simulink model "reduce_spect"  (R2013b)
settings: Solver=ode45  StartTime=0.0  StopTime=10.0  RelTol=1e-3
undefined symbols (not defined in the file): pfb_coeff_gen_calc
libraries: xbsIndex_r4 x15467, casper_library_delays x101, casper_library_misc x85, dspsigops x16, xps_library x4, xbsReplacements_r4 x2, casper_library_pfbs x2
(part 6 of 157)

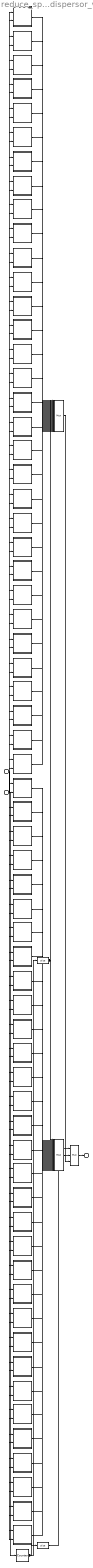
== system reduce_spect/Dedispersor_v4 ==
  Data : Inport
  Valid : Inport  Port=2
  Counter : xbsIndex_r4/Counter  cnt_type=Free Running  cnt_to=Inf  operation=Up  start_count=0  cnt_by_val=1  arith_type=Unsigned  n_bits=6  bin_pt=0  load_pin=off  rst=off  en=on  explicit_period=on  period=1  dbl_ovrd=off  use_behavioral_HDL=off  implementation=Fabric  block_type=counter
  Mux : xbsIndex_r4/Mux  inputs=32  en=off  latency=0  precision=Full  arith_type=Unsigned  n_bits=16  bin_pt=14  quantization=Truncate  overflow=Wrap  dbl_ovrd=off  block_type=mux
  Mux1 : xbsIndex_r4/Mux  inputs=32  en=off  latency=0  precision=Full  arith_type=Unsigned  n_bits=16  bin_pt=14  quantization=Truncate  overflow=Wrap  dbl_ovrd=off  block_type=mux
  Mux2 : xbsIndex_r4/Mux  inputs=2  en=off  latency=0  precision=Full  arith_type=Unsigned  n_bits=16  bin_pt=14  quantization=Truncate  overflow=Wrap  dbl_ovrd=off  block_type=mux
  Slice : xbsIndex_r4/Slice  nbits=5  boolean_output=off  mode=Lower Bit Location + Width  bit1=0  base1=MSB of Input  bit0=0  base0=LSB of Input  dbl_ovrd=off  block_type=slice
  Slice1 : xbsIndex_r4/Slice  nbits=1  boolean_output=off  mode=Upper Bit Location + Width  bit1=0  base1=MSB of Input  bit0=0  base0=LSB of Input  dbl_ovrd=off  block_type=slice
  detector_block_v2 : Subsystem  AncestorBlock=honestlibrary/detector_block_v2  mask(Basic block for FRB detection){chn=0, lat=1, nbits=6, behavioral=on}
      mask prompts: chn "Channel"; lat "Latency"; nbits "Number of Bits (Counter)"; behavioral "behavioral delay"
      mask help:
      | Delays a certain channel a number of latency clock cycles, according to the fixed DM table.
      | This version incorporates an internal counter (nbits) to know when store or give a certain value.
      mask init:
      | detector_block_init_v2(gcb,'chn',chn,'lat',lat,'nbits',nbits,'behavioral', behavioral)
      settings: AttributesFormatString=Channel: 0, Delay: 1
  detector_block_v21 : Subsystem  AncestorBlock=honestlibrary/detector_block_v2  mask(Basic block for FRB detection){chn=1, lat=2, nbits=6, behavioral=on}
      mask prompts: chn "Channel"; lat "Latency"; nbits "Number of Bits (Counter)"; behavioral "behavioral delay"
      mask help:
      | Delays a certain channel a number of latency clock cycles, according to the fixed DM table.
      | This version incorporates an internal counter (nbits) to know when store or give a certain value.
      mask init:
      | detector_block_init_v2(gcb,'chn',chn,'lat',lat,'nbits',nbits,'behavioral', behavioral)
      settings: AttributesFormatString=Channel: 1, Delay: 2
  detector_block_v210 : Subsystem  AncestorBlock=honestlibrary/detector_block_v2  mask(Basic block for FRB detection){chn=10, lat=29, nbits=6, behavioral=on}
      mask prompts: chn "Channel"; lat "Latency"; nbits "Number of Bits (Counter)"; behavioral "behavioral delay"
      mask help:
      | Delays a certain channel a number of latency clock cycles, according to the fixed DM table.
      | This version incorporates an internal counter (nbits) to know when store or give a certain value.
      mask init:
      | detector_block_init_v2(gcb,'chn',chn,'lat',lat,'nbits',nbits,'behavioral', behavioral)
      settings: AttributesFormatString=Channel: 10, Delay: 29
  detector_block_v211 : Subsystem  AncestorBlock=honestlibrary/detector_block_v2  mask(Basic block for FRB detection){chn=11, lat=31, nbits=6, behavioral=on}
      mask prompts: chn "Channel"; lat "Latency"; nbits "Number of Bits (Counter)"; behavioral "behavioral delay"
      mask help:
      | Delays a certain channel a number of latency clock cycles, according to the fixed DM table.
      | This version incorporates an internal counter (nbits) to know when store or give a certain value.
      mask init:
      | detector_block_init_v2(gcb,'chn',chn,'lat',lat,'nbits',nbits,'behavioral', behavioral)
      settings: AttributesFormatString=Channel: 11, Delay: 31
  detector_block_v212 : Subsystem  AncestorBlock=honestlibrary/detector_block_v2  mask(Basic block for FRB detection){chn=12, lat=34, nbits=6, behavioral=on}
      mask prompts: chn "Channel"; lat "Latency"; nbits "Number of Bits (Counter)"; behavioral "behavioral delay"
      mask help:
      | Delays a certain channel a number of latency clock cycles, according to the fixed DM table.
      | This version incorporates an internal counter (nbits) to know when store or give a certain value.
      mask init:
      | detector_block_init_v2(gcb,'chn',chn,'lat',lat,'nbits',nbits,'behavioral', behavioral)
      settings: AttributesFormatString=Channel: 12, Delay: 34
  detector_block_v213 : Subsystem  AncestorBlock=honestlibrary/detector_block_v2  mask(Basic block for FRB detection){chn=13, lat=37, nbits=6, behavioral=on}
      mask prompts: chn "Channel"; lat "Latency"; nbits "Number of Bits (Counter)"; behavioral "behavioral delay"
      mask help:
      | Delays a certain channel a number of latency clock cycles, according to the fixed DM table.
      | This version incorporates an internal counter (nbits) to know when store or give a certain value.
      mask init:
      | detector_block_init_v2(gcb,'chn',chn,'lat',lat,'nbits',nbits,'behavioral', behavioral)
      settings: AttributesFormatString=Channel: 13, Delay: 37
  detector_block_v214 : Subsystem  AncestorBlock=honestlibrary/detector_block_v2  mask(Basic block for FRB detection){chn=14, lat=39, nbits=6, behavioral=on}
      mask prompts: chn "Channel"; lat "Latency"; nbits "Number of Bits (Counter)"; behavioral "behavioral delay"
      mask help:
      | Delays a certain channel a number of latency clock cycles, according to the fixed DM table.
      | This version incorporates an internal counter (nbits) to know when store or give a certain value.
      mask init:
      | detector_block_init_v2(gcb,'chn',chn,'lat',lat,'nbits',nbits,'behavioral', behavioral)
      settings: AttributesFormatString=Channel: 14, Delay: 39
  detector_block_v215 : Subsystem  AncestorBlock=honestlibrary/detector_block_v2  mask(Basic block for FRB detection){chn=15, lat=41, nbits=6, behavioral=on}
      mask prompts: chn "Channel"; lat "Latency"; nbits "Number of Bits (Counter)"; behavioral "behavioral delay"
      mask help:
      | Delays a certain channel a number of latency clock cycles, according to the fixed DM table.
      | This version incorporates an internal counter (nbits) to know when store or give a certain value.
      mask init:
      | detector_block_init_v2(gcb,'chn',chn,'lat',lat,'nbits',nbits,'behavioral', behavioral)
      settings: AttributesFormatString=Channel: 15, Delay: 41
  detector_block_v216 : Subsystem  AncestorBlock=honestlibrary/detector_block_v2  mask(Basic block for FRB detection){chn=16, lat=44, nbits=6, behavioral=on}
      mask prompts: chn "Channel"; lat "Latency"; nbits "Number of Bits (Counter)"; behavioral "behavioral delay"
      mask help:
      | Delays a certain channel a number of latency clock cycles, according to the fixed DM table.
      | This version incorporates an internal counter (nbits) to know when store or give a certain value.
      mask init:
      | detector_block_init_v2(gcb,'chn',chn,'lat',lat,'nbits',nbits,'behavioral', behavioral)
      settings: AttributesFormatString=Channel: 16, Delay: 44
  detector_block_v217 : Subsystem  AncestorBlock=honestlibrary/detector_block_v2  mask(Basic block for FRB detection){chn=17, lat=46, nbits=6, behavioral=on}
      mask prompts: chn "Channel"; lat "Latency"; nbits "Number of Bits (Counter)"; behavioral "behavioral delay"
      mask help:
      | Delays a certain channel a number of latency clock cycles, according to the fixed DM table.
      | This version incorporates an internal counter (nbits) to know when store or give a certain value.
      mask init:
      | detector_block_init_v2(gcb,'chn',chn,'lat',lat,'nbits',nbits,'behavioral', behavioral)
      settings: AttributesFormatString=Channel: 17, Delay: 46
  detector_block_v218 : Subsystem  AncestorBlock=honestlibrary/detector_block_v2  mask(Basic block for FRB detection){chn=18, lat=48, nbits=6, behavioral=on}
      mask prompts: chn "Channel"; lat "Latency"; nbits "Number of Bits (Counter)"; behavioral "behavioral delay"
      mask help:
      | Delays a certain channel a number of latency clock cycles, according to the fixed DM table.
      | This version incorporates an internal counter (nbits) to know when store or give a certain value.
      mask init:
      | detector_block_init_v2(gcb,'chn',chn,'lat',lat,'nbits',nbits,'behavioral', behavioral)
      settings: AttributesFormatString=Channel: 18, Delay: 48
  detector_block_v219 : Subsystem  AncestorBlock=honestlibrary/detector_block_v2  mask(Basic block for FRB detection){chn=19, lat=51, nbits=6, behavioral=on}
      mask prompts: chn "Channel"; lat "Latency"; nbits "Number of Bits (Counter)"; behavioral "behavioral delay"
      mask help:
      | Delays a certain channel a number of latency clock cycles, according to the fixed DM table.
      | This version incorporates an internal counter (nbits) to know when store or give a certain value.
      mask init:
      | detector_block_init_v2(gcb,'chn',chn,'lat',lat,'nbits',nbits,'behavioral', behavioral)
      settings: AttributesFormatString=Channel: 19, Delay: 51
  detector_block_v22 : Subsystem  AncestorBlock=honestlibrary/detector_block_v2  mask(Basic block for FRB detection){chn=2, lat=5, nbits=6, behavioral=on}
      mask prompts: chn "Channel"; lat "Latency"; nbits "Number of Bits (Counter)"; behavioral "behavioral delay"
      mask help:
      | Delays a certain channel a number of latency clock cycles, according to the fixed DM table.
      | This version incorporates an internal counter (nbits) to know when store or give a certain value.
      mask init:
      | detector_block_init_v2(gcb,'chn',chn,'lat',lat,'nbits',nbits,'behavioral', behavioral)
      settings: AttributesFormatString=Channel: 2, Delay: 5
  detector_block_v220 : Subsystem  AncestorBlock=honestlibrary/detector_block_v2  mask(Basic block for FRB detection){chn=20, lat=53, nbits=6, behavioral=on}
      mask prompts: chn "Channel"; lat "Latency"; nbits "Number of Bits (Counter)"; behavioral "behavioral delay"
      mask help:
      | Delays a certain channel a number of latency clock cycles, according to the fixed DM table.
      | This version incorporates an internal counter (nbits) to know when store or give a certain value.
      mask init:
      | detector_block_init_v2(gcb,'chn',chn,'lat',lat,'nbits',nbits,'behavioral', behavioral)
      settings: AttributesFormatString=Channel: 20, Delay: 53
  detector_block_v221 : Subsystem  AncestorBlock=honestlibrary/detector_block_v2  mask(Basic block for FRB detection){chn=21, lat=55, nbits=6, behavioral=on}
      mask prompts: chn "Channel"; lat "Latency"; nbits "Number of Bits (Counter)"; behavioral "behavioral delay"
      mask help:
      | Delays a certain channel a number of latency clock cycles, according to the fixed DM table.
      | This version incorporates an internal counter (nbits) to know when store or give a certain value.
      mask init:
      | detector_block_init_v2(gcb,'chn',chn,'lat',lat,'nbits',nbits,'behavioral', behavioral)
      settings: AttributesFormatString=Channel: 21, Delay: 55
  detector_block_v222 : Subsystem  AncestorBlock=honestlibrary/detector_block_v2  mask(Basic block for FRB detection){chn=22, lat=57, nbits=6, behavioral=on}
      mask prompts: chn "Channel"; lat "Latency"; nbits "Number of Bits (Counter)"; behavioral "behavioral delay"
      mask help:
      | Delays a certain channel a number of latency clock cycles, according to the fixed DM table.
      | This version incorporates an internal counter (nbits) to know when store or give a certain value.
      mask init:
      | detector_block_init_v2(gcb,'chn',chn,'lat',lat,'nbits',nbits,'behavioral', behavioral)
      settings: AttributesFormatString=Channel: 22, Delay: 57
  detector_block_v223 : Subsystem  AncestorBlock=honestlibrary/detector_block_v2  mask(Basic block for FRB detection){chn=23, lat=59, nbits=6, behavioral=on}
      mask prompts: chn "Channel"; lat "Latency"; nbits "Number of Bits (Counter)"; behavioral "behavioral delay"
      mask help:
      | Delays a certain channel a number of latency clock cycles, according to the fixed DM table.
      | This version incorporates an internal counter (nbits) to know when store or give a certain value.
      mask init:
      | detector_block_init_v2(gcb,'chn',chn,'lat',lat,'nbits',nbits,'behavioral', behavioral)
      settings: AttributesFormatString=Channel: 23, Delay: 59
  detector_block_v224 : Subsystem  AncestorBlock=honestlibrary/detector_block_v2  mask(Basic block for FRB detection){chn=24, lat=61, nbits=6, behavioral=on}
      mask prompts: chn "Channel"; lat "Latency"; nbits "Number of Bits (Counter)"; behavioral "behavioral delay"
      mask help:
      | Delays a certain channel a number of latency clock cycles, according to the fixed DM table.
      | This version incorporates an internal counter (nbits) to know when store or give a certain value.
      mask init:
      | detector_block_init_v2(gcb,'chn',chn,'lat',lat,'nbits',nbits,'behavioral', behavioral)
      settings: AttributesFormatString=Channel: 24, Delay: 61
  detector_block_v225 : Subsystem  AncestorBlock=honestlibrary/detector_block_v2  mask(Basic block for FRB detection){chn=25, lat=63, nbits=6, behavioral=on}
      mask prompts: chn "Channel"; lat "Latency"; nbits "Number of Bits (Counter)"; behavioral "behavioral delay"
      mask help:
      | Delays a certain channel a number of latency clock cycles, according to the fixed DM table.
      | This version incorporates an internal counter (nbits) to know when store or give a certain value.
      mask init:
      | detector_block_init_v2(gcb,'chn',chn,'lat',lat,'nbits',nbits,'behavioral', behavioral)
      settings: AttributesFormatString=Channel: 25, Delay: 63
  detector_block_v226 : Subsystem  AncestorBlock=honestlibrary/detector_block_v2  mask(Basic block for FRB detection){chn=26, lat=65, nbits=6, behavioral=on}
      mask prompts: chn "Channel"; lat "Latency"; nbits "Number of Bits (Counter)"; behavioral "behavioral delay"
      mask help:
      | Delays a certain channel a number of latency clock cycles, according to the fixed DM table.
      | This version incorporates an internal counter (nbits) to know when store or give a certain value.
      mask init:
      | detector_block_init_v2(gcb,'chn',chn,'lat',lat,'nbits',nbits,'behavioral', behavioral)
      settings: AttributesFormatString=Channel: 26, Delay: 65
  detector_block_v227 : Subsystem  AncestorBlock=honestlibrary/detector_block_v2  mask(Basic block for FRB detection){chn=27, lat=67, nbits=6, behavioral=on}
      mask prompts: chn "Channel"; lat "Latency"; nbits "Number of Bits (Counter)"; behavioral "behavioral delay"
      mask help:
      | Delays a certain channel a number of latency clock cycles, according to the fixed DM table.
      | This version incorporates an internal counter (nbits) to know when store or give a certain value.
      mask init:
      | detector_block_init_v2(gcb,'chn',chn,'lat',lat,'nbits',nbits,'behavioral', behavioral)
      settings: AttributesFormatString=Channel: 27, Delay: 67
  detector_block_v228 : Subsystem  AncestorBlock=honestlibrary/detector_block_v2  mask(Basic block for FRB detection){chn=28, lat=69, nbits=6, behavioral=on}
      mask prompts: chn "Channel"; lat "Latency"; nbits "Number of Bits (Counter)"; behavioral "behavioral delay"
      mask help:
      | Delays a certain channel a number of latency clock cycles, according to the fixed DM table.
      | This version incorporates an internal counter (nbits) to know when store or give a certain value.
      mask init:
      | detector_block_init_v2(gcb,'chn',chn,'lat',lat,'nbits',nbits,'behavioral', behavioral)
      settings: AttributesFormatString=Channel: 28, Delay: 69
  detector_block_v229 : Subsystem  AncestorBlock=honestlibrary/detector_block_v2  mask(Basic block for FRB detection){chn=29, lat=71, nbits=6, behavioral=on}
      mask prompts: chn "Channel"; lat "Latency"; nbits "Number of Bits (Counter)"; behavioral "behavioral delay"
      mask help:
      | Delays a certain channel a number of latency clock cycles, according to the fixed DM table.
      | This version incorporates an internal counter (nbits) to know when store or give a certain value.
      mask init:
      | detector_block_init_v2(gcb,'chn',chn,'lat',lat,'nbits',nbits,'behavioral', behavioral)
      settings: AttributesFormatString=Channel: 29, Delay: 71
  detector_block_v23 : Subsystem  AncestorBlock=honestlibrary/detector_block_v2  mask(Basic block for FRB detection){chn=3, lat=8, nbits=6, behavioral=on}
      mask prompts: chn "Channel"; lat "Latency"; nbits "Number of Bits (Counter)"; behavioral "behavioral delay"
      mask help:
      | Delays a certain channel a number of latency clock cycles, according to the fixed DM table.
      | This version incorporates an internal counter (nbits) to know when store or give a certain value.
      mask init:
      | detector_block_init_v2(gcb,'chn',chn,'lat',lat,'nbits',nbits,'behavioral', behavioral)
      settings: AttributesFormatString=Channel: 3, Delay: 8
  detector_block_v230 : Subsystem  AncestorBlock=honestlibrary/detector_block_v2  mask(Basic block for FRB detection){chn=30, lat=73, nbits=6, behavioral=on}
      mask prompts: chn "Channel"; lat "Latency"; nbits "Number of Bits (Counter)"; behavioral "behavioral delay"
      mask help:
      | Delays a certain channel a number of latency clock cycles, according to the fixed DM table.
      | This version incorporates an internal counter (nbits) to know when store or give a certain value.
      mask init:
      | detector_block_init_v2(gcb,'chn',chn,'lat',lat,'nbits',nbits,'behavioral', behavioral)
      settings: AttributesFormatString=Channel: 30, Delay: 73
  detector_block_v231 : Subsystem  AncestorBlock=honestlibrary/detector_block_v2  mask(Basic block for FRB detection){chn=31, lat=74, nbits=6, behavioral=on}
      mask prompts: chn "Channel"; lat "Latency"; nbits "Number of Bits (Counter)"; behavioral "behavioral delay"
      mask help:
      | Delays a certain channel a number of latency clock cycles, according to the fixed DM table.
      | This version incorporates an internal counter (nbits) to know when store or give a certain value.
      mask init:
      | detector_block_init_v2(gcb,'chn',chn,'lat',lat,'nbits',nbits,'behavioral', behavioral)
      settings: AttributesFormatString=Channel: 31, Delay: 74
  detector_block_v232 : Subsystem  AncestorBlock=honestlibrary/detector_block_v2  mask(Basic block for FRB detection){chn=32, lat=76, nbits=6, behavioral=on}
      mask prompts: chn "Channel"; lat "Latency"; nbits "Number of Bits (Counter)"; behavioral "behavioral delay"
      mask help:
      | Delays a certain channel a number of latency clock cycles, according to the fixed DM table.
      | This version incorporates an internal counter (nbits) to know when store or give a certain value.
      mask init:
      | detector_block_init_v2(gcb,'chn',chn,'lat',lat,'nbits',nbits,'behavioral', behavioral)
      settings: AttributesFormatString=Channel: 32, Delay: 76
  detector_block_v233 : Subsystem  AncestorBlock=honestlibrary/detector_block_v2  mask(Basic block for FRB detection){chn=33, lat=78, nbits=6, behavioral=on}
      mask prompts: chn "Channel"; lat "Latency"; nbits "Number of Bits (Counter)"; behavioral "behavioral delay"
      mask help:
      | Delays a certain channel a number of latency clock cycles, according to the fixed DM table.
      | This version incorporates an internal counter (nbits) to know when store or give a certain value.
      mask init:
      | detector_block_init_v2(gcb,'chn',chn,'lat',lat,'nbits',nbits,'behavioral', behavioral)
      settings: AttributesFormatString=Channel: 33, Delay: 78
  detector_block_v234 : Subsystem  AncestorBlock=honestlibrary/detector_block_v2  mask(Basic block for FRB detection){chn=34, lat=79, nbits=6, behavioral=on}
      mask prompts: chn "Channel"; lat "Latency"; nbits "Number of Bits (Counter)"; behavioral "behavioral delay"
      mask help:
      | Delays a certain channel a number of latency clock cycles, according to the fixed DM table.
      | This version incorporates an internal counter (nbits) to know when store or give a certain value.
      mask init:
      | detector_block_init_v2(gcb,'chn',chn,'lat',lat,'nbits',nbits,'behavioral', behavioral)
      settings: AttributesFormatString=Channel: 34, Delay: 79
  detector_block_v235 : Subsystem  AncestorBlock=honestlibrary/detector_block_v2  mask(Basic block for FRB detection){chn=35, lat=81, nbits=6, behavioral=on}
      mask prompts: chn "Channel"; lat "Latency"; nbits "Number of Bits (Counter)"; behavioral "behavioral delay"
      mask help:
      | Delays a certain channel a number of latency clock cycles, according to the fixed DM table.
      | This version incorporates an internal counter (nbits) to know when store or give a certain value.
      mask init:
      | detector_block_init_v2(gcb,'chn',chn,'lat',lat,'nbits',nbits,'behavioral', behavioral)
      settings: AttributesFormatString=Channel: 35, Delay: 81
  detector_block_v236 : Subsystem  AncestorBlock=honestlibrary/detector_block_v2  mask(Basic block for FRB detection){chn=36, lat=83, nbits=6, behavioral=on}
      mask prompts: chn "Channel"; lat "Latency"; nbits "Number of Bits (Counter)"; behavioral "behavioral delay"
      mask help:
      | Delays a certain channel a number of latency clock cycles, according to the fixed DM table.
      | This version incorporates an internal counter (nbits) to know when store or give a certain value.
      mask init:
      | detector_block_init_v2(gcb,'chn',chn,'lat',lat,'nbits',nbits,'behavioral', behavioral)
      settings: AttributesFormatString=Channel: 36, Delay: 83
  detector_block_v237 : Subsystem  AncestorBlock=honestlibrary/detector_block_v2  mask(Basic block for FRB detection){chn=37, lat=84, nbits=6, behavioral=on}
      mask prompts: chn "Channel"; lat "Latency"; nbits "Number of Bits (Counter)"; behavioral "behavioral delay"
      mask help:
      | Delays a certain channel a number of latency clock cycles, according to the fixed DM table.
      | This version incorporates an internal counter (nbits) to know when store or give a certain value.
      mask init:
      | detector_block_init_v2(gcb,'chn',chn,'lat',lat,'nbits',nbits,'behavioral', behavioral)
      settings: AttributesFormatString=Channel: 37, Delay: 84
  detector_block_v238 : Subsystem  AncestorBlock=honestlibrary/detector_block_v2  mask(Basic block for FRB detection){chn=38, lat=86, nbits=6, behavioral=on}
      mask prompts: chn "Channel"; lat "Latency"; nbits "Number of Bits (Counter)"; behavioral "behavioral delay"
      mask help:
      | Delays a certain channel a number of latency clock cycles, according to the fixed DM table.
      | This version incorporates an internal counter (nbits) to know when store or give a certain value.
      mask init:
      | detector_block_init_v2(gcb,'chn',chn,'lat',lat,'nbits',nbits,'behavioral', behavioral)
      settings: AttributesFormatString=Channel: 38, Delay: 86
  detector_block_v239 : Subsystem  AncestorBlock=honestlibrary/detector_block_v2  mask(Basic block for FRB detection){chn=39, lat=87, nbits=6, behavioral=on}
      mask prompts: chn "Channel"; lat "Latency"; nbits "Number of Bits (Counter)"; behavioral "behavioral delay"
      mask help:
      | Delays a certain channel a number of latency clock cycles, according to the fixed DM table.
      | This version incorporates an internal counter (nbits) to know when store or give a certain value.
      mask init:
      | detector_block_init_v2(gcb,'chn',chn,'lat',lat,'nbits',nbits,'behavioral', behavioral)
      settings: AttributesFormatString=Channel: 39, Delay: 87
  detector_block_v24 : Subsystem  AncestorBlock=honestlibrary/detector_block_v2  mask(Basic block for FRB detection){chn=4, lat=12, nbits=6, behavioral=on}
      mask prompts: chn "Channel"; lat "Latency"; nbits "Number of Bits (Counter)"; behavioral "behavioral delay"
      mask help:
      | Delays a certain channel a number of latency clock cycles, according to the fixed DM table.
      | This version incorporates an internal counter (nbits) to know when store or give a certain value.
      mask init:
      | detector_block_init_v2(gcb,'chn',chn,'lat',lat,'nbits',nbits,'behavioral', behavioral)
      settings: AttributesFormatString=Channel: 4, Delay: 12
  detector_block_v240 : Subsystem  AncestorBlock=honestlibrary/detector_block_v2  mask(Basic block for FRB detection){chn=40, lat=89, nbits=6, behavioral=on}
      mask prompts: chn "Channel"; lat "Latency"; nbits "Number of Bits (Counter)"; behavioral "behavioral delay"
      mask help:
      | Delays a certain channel a number of latency clock cycles, according to the fixed DM table.
      | This version incorporates an internal counter (nbits) to know when store or give a certain value.
      mask init:
      | detector_block_init_v2(gcb,'chn',chn,'lat',lat,'nbits',nbits,'behavioral', behavioral)
      settings: AttributesFormatString=Channel: 40, Delay: 89
  detector_block_v241 : Subsystem  AncestorBlock=honestlibrary/detector_block_v2  mask(Basic block for FRB detection){chn=41, lat=90, nbits=6, behavioral=on}
      mask prompts: chn "Channel"; lat "Latency"; nbits "Number of Bits (Counter)"; behavioral "behavioral delay"
      mask help:
      | Delays a certain channel a number of latency clock cycles, according to the fixed DM table.
      | This version incorporates an internal counter (nbits) to know when store or give a certain value.
      mask init:
      | detector_block_init_v2(gcb,'chn',chn,'lat',lat,'nbits',nbits,'behavioral', behavioral)
      settings: AttributesFormatString=Channel: 41, Delay: 90
  detector_block_v242 : Subsystem  AncestorBlock=honestlibrary/detector_block_v2  mask(Basic block for FRB detection){chn=42, lat=92, nbits=6, behavioral=on}
      mask prompts: chn "Channel"; lat "Latency"; nbits "Number of Bits (Counter)"; behavioral "behavioral delay"
      mask help:
      | Delays a certain channel a number of latency clock cycles, according to the fixed DM table.
      | This version incorporates an internal counter (nbits) to know when store or give a certain value.
      mask init:
      | detector_block_init_v2(gcb,'chn',chn,'lat',lat,'nbits',nbits,'behavioral', behavioral)
      settings: AttributesFormatString=Channel: 42, Delay: 92
  detector_block_v243 : Subsystem  AncestorBlock=honestlibrary/detector_block_v2  mask(Basic block for FRB detection){chn=43, lat=93, nbits=6, behavioral=on}
      mask prompts: chn "Channel"; lat "Latency"; nbits "Number of Bits (Counter)"; behavioral "behavioral delay"
      mask help:
      | Delays a certain channel a number of latency clock cycles, according to the fixed DM table.
      | This version incorporates an internal counter (nbits) to know when store or give a certain value.
      mask init:
      | detector_block_init_v2(gcb,'chn',chn,'lat',lat,'nbits',nbits,'behavioral', behavioral)
      settings: AttributesFormatString=Channel: 43, Delay: 93
  detector_block_v244 : Subsystem  AncestorBlock=honestlibrary/detector_block_v2  mask(Basic block for FRB detection){chn=44, lat=95, nbits=6, behavioral=on}
      mask prompts: chn "Channel"; lat "Latency"; nbits "Number of Bits (Counter)"; behavioral "behavioral delay"
      mask help:
      | Delays a certain channel a number of latency clock cycles, according to the fixed DM table.
      | This version incorporates an internal counter (nbits) to know when store or give a certain value.
      mask init:
      | detector_block_init_v2(gcb,'chn',chn,'lat',lat,'nbits',nbits,'behavioral', behavioral)
      settings: AttributesFormatString=Channel: 44, Delay: 95
  detector_block_v245 : Subsystem  AncestorBlock=honestlibrary/detector_block_v2  mask(Basic block for FRB detection){chn=45, lat=96, nbits=6, behavioral=on}
      mask prompts: chn "Channel"; lat "Latency"; nbits "Number of Bits (Counter)"; behavioral "behavioral delay"
      mask help:
      | Delays a certain channel a number of latency clock cycles, according to the fixed DM table.
      | This version incorporates an internal counter (nbits) to know when store or give a certain value.
      mask init:
      | detector_block_init_v2(gcb,'chn',chn,'lat',lat,'nbits',nbits,'behavioral', behavioral)
      settings: AttributesFormatString=Channel: 45, Delay: 96
  detector_block_v246 : Subsystem  AncestorBlock=honestlibrary/detector_block_v2  mask(Basic block for FRB detection){chn=46, lat=97, nbits=6, behavioral=on}
      mask prompts: chn "Channel"; lat "Latency"; nbits "Number of Bits (Counter)"; behavioral "behavioral delay"
      mask help:
      | Delays a certain channel a number of latency clock cycles, according to the fixed DM table.
      | This version incorporates an internal counter (nbits) to know when store or give a certain value.
      mask init:
      | detector_block_init_v2(gcb,'chn',chn,'lat',lat,'nbits',nbits,'behavioral', behavioral)
      settings: AttributesFormatString=Channel: 46, Delay: 97
  detector_block_v247 : Subsystem  AncestorBlock=honestlibrary/detector_block_v2  mask(Basic block for FRB detection){chn=47, lat=99, nbits=6, behavioral=on}
      mask prompts: chn "Channel"; lat "Latency"; nbits "Number of Bits (Counter)"; behavioral "behavioral delay"
      mask help:
      | Delays a certain channel a number of latency clock cycles, according to the fixed DM table.
      | This version incorporates an internal counter (nbits) to know when store or give a certain value.
      mask init:
      | detector_block_init_v2(gcb,'chn',chn,'lat',lat,'nbits',nbits,'behavioral', behavioral)
      settings: AttributesFormatString=Channel: 47, Delay: 99
  detector_block_v248 : Subsystem  AncestorBlock=honestlibrary/detector_block_v2  mask(Basic block for FRB detection){chn=48, lat=100, nbits=6, behavioral=on}
      mask prompts: chn "Channel"; lat "Latency"; nbits "Number of Bits (Counter)"; behavioral "behavioral delay"
      mask help:
      | Delays a certain channel a number of latency clock cycles, according to the fixed DM table.
      | This version incorporates an internal counter (nbits) to know when store or give a certain value.
      mask init:
      | detector_block_init_v2(gcb,'chn',chn,'lat',lat,'nbits',nbits,'behavioral', behavioral)
      settings: AttributesFormatString=Channel: 48, Delay: 100
  detector_block_v249 : Subsystem  AncestorBlock=honestlibrary/detector_block_v2  mask(Basic block for FRB detection){chn=49, lat=101, nbits=6, behavioral=on}
      mask prompts: chn "Channel"; lat "Latency"; nbits "Number of Bits (Counter)"; behavioral "behavioral delay"
      mask help:
      | Delays a certain channel a number of latency clock cycles, according to the fixed DM table.
      | This version incorporates an internal counter (nbits) to know when store or give a certain value.
      mask init:
      | detector_block_init_v2(gcb,'chn',chn,'lat',lat,'nbits',nbits,'behavioral', behavioral)
      settings: AttributesFormatString=Channel: 49, Delay: 101
  detector_block_v25 : Subsystem  AncestorBlock=honestlibrary/detector_block_v2  mask(Basic block for FRB detection){chn=5, lat=15, nbits=6, behavioral=on}
      mask prompts: chn "Channel"; lat "Latency"; nbits "Number of Bits (Counter)"; behavioral "behavioral delay"
      mask help:
      | Delays a certain channel a number of latency clock cycles, according to the fixed DM table.
      | This version incorporates an internal counter (nbits) to know when store or give a certain value.
      mask init:
      | detector_block_init_v2(gcb,'chn',chn,'lat',lat,'nbits',nbits,'behavioral', behavioral)
      settings: AttributesFormatString=Channel: 5, Delay: 15
  detector_block_v250 : Subsystem  AncestorBlock=honestlibrary/detector_block_v2  mask(Basic block for FRB detection){chn=50, lat=102, nbits=6, behavioral=on}
      mask prompts: chn "Channel"; lat "Latency"; nbits "Number of Bits (Counter)"; behavioral "behavioral delay"
      mask help:
      | Delays a certain channel a number of latency clock cycles, according to the fixed DM table.
      | This version incorporates an internal counter (nbits) to know when store or give a certain value.
      mask init:
      | detector_block_init_v2(gcb,'chn',chn,'lat',lat,'nbits',nbits,'behavioral', behavioral)
      settings: AttributesFormatString=Channel: 50, Delay: 102
  detector_block_v251 : Subsystem  AncestorBlock=honestlibrary/detector_block_v2  mask(Basic block for FRB detection){chn=51, lat=104, nbits=6, behavioral=on}
      mask prompts: chn "Channel"; lat "Latency"; nbits "Number of Bits (Counter)"; behavioral "behavioral delay"
      mask help:
      | Delays a certain channel a number of latency clock cycles, according to the fixed DM table.
      | This version incorporates an internal counter (nbits) to know when store or give a certain value.
      mask init:
      | detector_block_init_v2(gcb,'chn',chn,'lat',lat,'nbits',nbits,'behavioral', behavioral)
      settings: AttributesFormatString=Channel: 51, Delay: 104
  detector_block_v252 : Subsystem  AncestorBlock=honestlibrary/detector_block_v2  mask(Basic block for FRB detection){chn=52, lat=105, nbits=6, behavioral=on}
      mask prompts: chn "Channel"; lat "Latency"; nbits "Number of Bits (Counter)"; behavioral "behavioral delay"
      mask help:
      | Delays a certain channel a number of latency clock cycles, according to the fixed DM table.
      | This version incorporates an internal counter (nbits) to know when store or give a certain value.
      mask init:
      | detector_block_init_v2(gcb,'chn',chn,'lat',lat,'nbits',nbits,'behavioral', behavioral)
      settings: AttributesFormatString=Channel: 52, Delay: 105
  detector_block_v253 : Subsystem  AncestorBlock=honestlibrary/detector_block_v2  mask(Basic block for FRB detection){chn=53, lat=106, nbits=6, behavioral=on}
      mask prompts: chn "Channel"; lat "Latency"; nbits "Number of Bits (Counter)"; behavioral "behavioral delay"
      mask help:
      | Delays a certain channel a number of latency clock cycles, according to the fixed DM table.
      | This version incorporates an internal counter (nbits) to know when store or give a certain value.
      mask init:
      | detector_block_init_v2(gcb,'chn',chn,'lat',lat,'nbits',nbits,'behavioral', behavioral)
      settings: AttributesFormatString=Channel: 53, Delay: 106
  detector_block_v254 : Subsystem  AncestorBlock=honestlibrary/detector_block_v2  mask(Basic block for FRB detection){chn=54, lat=107, nbits=6, behavioral=on}
      mask prompts: chn "Channel"; lat "Latency"; nbits "Number of Bits (Counter)"; behavioral "behavioral delay"
      mask help:
      | Delays a certain channel a number of latency clock cycles, according to the fixed DM table.
      | This version incorporates an internal counter (nbits) to know when store or give a certain value.
      mask init:
      | detector_block_init_v2(gcb,'chn',chn,'lat',lat,'nbits',nbits,'behavioral', behavioral)
      settings: AttributesFormatString=Channel: 54, Delay: 107
  detector_block_v255 : Subsystem  AncestorBlock=honestlibrary/detector_block_v2  mask(Basic block for FRB detection){chn=55, lat=108, nbits=6, behavioral=on}
      mask prompts: chn "Channel"; lat "Latency"; nbits "Number of Bits (Counter)"; behavioral "behavioral delay"
      mask help:
      | Delays a certain channel a number of latency clock cycles, according to the fixed DM table.
      | This version incorporates an internal counter (nbits) to know when store or give a certain value.
      mask init:
      | detector_block_init_v2(gcb,'chn',chn,'lat',lat,'nbits',nbits,'behavioral', behavioral)
      settings: AttributesFormatString=Channel: 55, Delay: 108
  detector_block_v256 : Subsystem  AncestorBlock=honestlibrary/detector_block_v2  mask(Basic block for FRB detection){chn=56, lat=110, nbits=6, behavioral=on}
      mask prompts: chn "Channel"; lat "Latency"; nbits "Number of Bits (Counter)"; behavioral "behavioral delay"
      mask help:
      | Delays a certain channel a number of latency clock cycles, according to the fixed DM table.
      | This version incorporates an internal counter (nbits) to know when store or give a certain value.
      mask init:
      | detector_block_init_v2(gcb,'chn',chn,'lat',lat,'nbits',nbits,'behavioral', behavioral)
      settings: AttributesFormatString=Channel: 56, Delay: 110
  detector_block_v257 : Subsystem  AncestorBlock=honestlibrary/detector_block_v2  mask(Basic block for FRB detection){chn=57, lat=111, nbits=6, behavioral=on}
      mask prompts: chn "Channel"; lat "Latency"; nbits "Number of Bits (Counter)"; behavioral "behavioral delay"
      mask help:
      | Delays a certain channel a number of latency clock cycles, according to the fixed DM table.
      | This version incorporates an internal counter (nbits) to know when store or give a certain value.
      mask init:
      | detector_block_init_v2(gcb,'chn',chn,'lat',lat,'nbits',nbits,'behavioral', behavioral)
      settings: AttributesFormatString=Channel: 57, Delay: 111
  detector_block_v258 : Subsystem  AncestorBlock=honestlibrary/detector_block_v2  mask(Basic block for FRB detection){chn=58, lat=112, nbits=6, behavioral=on}
      mask prompts: chn "Channel"; lat "Latency"; nbits "Number of Bits (Counter)"; behavioral "behavioral delay"
      mask help:
      | Delays a certain channel a number of latency clock cycles, according to the fixed DM table.
      | This version incorporates an internal counter (nbits) to know when store or give a certain value.
      mask init:
      | detector_block_init_v2(gcb,'chn',chn,'lat',lat,'nbits',nbits,'behavioral', behavioral)
      settings: AttributesFormatString=Channel: 58, Delay: 112
  detector_block_v259 : Subsystem  AncestorBlock=honestlibrary/detector_block_v2  mask(Basic block for FRB detection){chn=59, lat=113, nbits=6, behavioral=on}
      mask prompts: chn "Channel"; lat "Latency"; nbits "Number of Bits (Counter)"; behavioral "behavioral delay"
      mask help:
      | Delays a certain channel a number of latency clock cycles, according to the fixed DM table.
      | This version incorporates an internal counter (nbits) to know when store or give a certain value.
      mask init:
      | detector_block_init_v2(gcb,'chn',chn,'lat',lat,'nbits',nbits,'behavioral', behavioral)
      settings: AttributesFormatString=Channel: 59, Delay: 113
  detector_block_v26 : Subsystem  AncestorBlock=honestlibrary/detector_block_v2  mask(Basic block for FRB detection){chn=6, lat=18, nbits=6, behavioral=on}
      mask prompts: chn "Channel"; lat "Latency"; nbits "Number of Bits (Counter)"; behavioral "behavioral delay"
      mask help:
      | Delays a certain channel a number of latency clock cycles, according to the fixed DM table.
      | This version incorporates an internal counter (nbits) to know when store or give a certain value.
      mask init:
      | detector_block_init_v2(gcb,'chn',chn,'lat',lat,'nbits',nbits,'behavioral', behavioral)
      settings: AttributesFormatString=Channel: 6, Delay: 18
  detector_block_v260 : Subsystem  AncestorBlock=honestlibrary/detector_block_v2  mask(Basic block for FRB detection){chn=60, lat=114, nbits=6, behavioral=on}
      mask prompts: chn "Channel"; lat "Latency"; nbits "Number of Bits (Counter)"; behavioral "behavioral delay"
      mask help:
      | Delays a certain channel a number of latency clock cycles, according to the fixed DM table.
      | This version incorporates an internal counter (nbits) to know when store or give a certain value.
      mask init:
      | detector_block_init_v2(gcb,'chn',chn,'lat',lat,'nbits',nbits,'behavioral', behavioral)
      settings: AttributesFormatString=Channel: 60, Delay: 114
  detector_block_v261 : Subsystem  AncestorBlock=honestlibrary/detector_block_v2  mask(Basic block for FRB detection){chn=61, lat=115, nbits=6, behavioral=on}
      mask prompts: chn "Channel"; lat "Latency"; nbits "Number of Bits (Counter)"; behavioral "behavioral delay"
      mask help:
      | Delays a certain channel a number of latency clock cycles, according to the fixed DM table.
      | This version incorporates an internal counter (nbits) to know when store or give a certain value.
      mask init:
      | detector_block_init_v2(gcb,'chn',chn,'lat',lat,'nbits',nbits,'behavioral', behavioral)
      settings: AttributesFormatString=Channel: 61, Delay: 115
  detector_block_v262 : Subsystem  AncestorBlock=honestlibrary/detector_block_v2  mask(Basic block for FRB detection){chn=62, lat=116, nbits=6, behavioral=on}
      mask prompts: chn "Channel"; lat "Latency"; nbits "Number of Bits (Counter)"; behavioral "behavioral delay"
      mask help:
      | Delays a certain channel a number of latency clock cycles, according to the fixed DM table.
      | This version incorporates an internal counter (nbits) to know when store or give a certain value.
      mask init:
      | detector_block_init_v2(gcb,'chn',chn,'lat',lat,'nbits',nbits,'behavioral', behavioral)
      settings: AttributesFormatString=Channel: 62, Delay: 116
  detector_block_v263 : Subsystem  AncestorBlock=honestlibrary/detector_block_v2  mask(Basic block for FRB detection){chn=63, lat=117, nbits=6, behavioral=on}
      mask prompts: chn "Channel"; lat "Latency"; nbits "Number of Bits (Counter)"; behavioral "behavioral delay"
      mask help:
      | Delays a certain channel a number of latency clock cycles, according to the fixed DM table.
      | This version incorporates an internal counter (nbits) to know when store or give a certain value.
      mask init:
      | detector_block_init_v2(gcb,'chn',chn,'lat',lat,'nbits',nbits,'behavioral', behavioral)
      settings: AttributesFormatString=Channel: 63, Delay: 117
  detector_block_v27 : Subsystem  AncestorBlock=honestlibrary/detector_block_v2  mask(Basic block for FRB detection){chn=7, lat=20, nbits=6, behavioral=on}
      mask prompts: chn "Channel"; lat "Latency"; nbits "Number of Bits (Counter)"; behavioral "behavioral delay"
      mask help:
      | Delays a certain channel a number of latency clock cycles, according to the fixed DM table.
      | This version incorporates an internal counter (nbits) to know when store or give a certain value.
      mask init:
      | detector_block_init_v2(gcb,'chn',chn,'lat',lat,'nbits',nbits,'behavioral', behavioral)
      settings: AttributesFormatString=Channel: 7, Delay: 20
  detector_block_v28 : Subsystem  AncestorBlock=honestlibrary/detector_block_v2  mask(Basic block for FRB detection){chn=8, lat=23, nbits=6, behavioral=on}
      mask prompts: chn "Channel"; lat "Latency"; nbits "Number of Bits (Counter)"; behavioral "behavioral delay"
      mask help:
      | Delays a certain channel a number of latency clock cycles, according to the fixed DM table.
      | This version incorporates an internal counter (nbits) to know when store or give a certain value.
      mask init:
      | detector_block_init_v2(gcb,'chn',chn,'lat',lat,'nbits',nbits,'behavioral', behavioral)
      settings: AttributesFormatString=Channel: 8, Delay: 23
  detector_block_v29 : Subsystem  AncestorBlock=honestlibrary/detector_block_v2  mask(Basic block for FRB detection){chn=9, lat=26, nbits=6, behavioral=on}
      mask prompts: chn "Channel"; lat "Latency"; nbits "Number of Bits (Counter)"; behavioral "behavioral delay"
      mask help:
      | Delays a certain channel a number of latency clock cycles, according to the fixed DM table.
      | This version incorporates an internal counter (nbits) to know when store or give a certain value.
      mask init:
      | detector_block_init_v2(gcb,'chn',chn,'lat',lat,'nbits',nbits,'behavioral', behavioral)
      settings: AttributesFormatString=Channel: 9, Delay: 26
  Output : Outport
  wires:
  Data/1 -> detector_block_v263/1(Data), detector_block_v262/1(Data), detector_block_v261/1(Data), detector_block_v260/1(Data), detector_block_v259/1(Data), detector_block_v258/1(Data), detector_block_v257/1(Data), detector_block_v256/1(Data), detector_block_v255/1(Data), detector_block_v254/1(Data), detector_block_v253/1(Data), detector_block_v252/1(Data), detector_block_v251/1(Data), detector_block_v250/1(Data), detector_block_v249/1(Data), detector_block_v248/1(Data), detector_block_v247/1(Data), detector_block_v246/1(Data), detector_block_v245/1(Data), detector_block_v244/1(Data), detector_block_v243/1(Data), detector_block_v242/1(Data), detector_block_v241/1(Data), detector_block_v240/1(Data), detector_block_v239/1(Data), detector_block_v238/1(Data), detector_block_v237/1(Data), detector_block_v236/1(Data), detector_block_v235/1(Data), detector_block_v234/1(Data), detector_block_v233/1(Data), detector_block_v232/1(Data), detector_block_v231/1(Data), detector_block_v230/1(Data), detector_block_v229/1(Data), detector_block_v228/1(Data), detector_block_v227/1(Data), detector_block_v226/1(Data), detector_block_v225/1(Data), detector_block_v224/1(Data), detector_block_v223/1(Data), detector_block_v222/1(Data), detector_block_v221/1(Data), detector_block_v220/1(Data), detector_block_v219/1(Data), detector_block_v218/1(Data), detector_block_v217/1(Data), detector_block_v216/1(Data), detector_block_v215/1(Data), detector_block_v214/1(Data), detector_block_v213/1(Data), detector_block_v212/1(Data), detector_block_v211/1(Data), detector_block_v210/1(Data), detector_block_v29/1(Data), detector_block_v28/1(Data), detector_block_v27/1(Data), detector_block_v26/1(Data), detector_block_v25/1(Data), detector_block_v24/1(Data), detector_block_v23/1(Data), detector_block_v22/1(Data), detector_block_v21/1(Data), detector_block_v2/1(Data)
  Valid/1 -> Counter/1, detector_block_v263/2(Valid), detector_block_v262/2(Valid), detector_block_v261/2(Valid), detector_block_v260/2(Valid), detector_block_v259/2(Valid), detector_block_v258/2(Valid), detector_block_v257/2(Valid), detector_block_v256/2(Valid), detector_block_v255/2(Valid), detector_block_v254/2(Valid), detector_block_v253/2(Valid), detector_block_v252/2(Valid), detector_block_v251/2(Valid), detector_block_v250/2(Valid), detector_block_v249/2(Valid), detector_block_v248/2(Valid), detector_block_v247/2(Valid), detector_block_v246/2(Valid), detector_block_v245/2(Valid), detector_block_v244/2(Valid), detector_block_v243/2(Valid), detector_block_v242/2(Valid), detector_block_v241/2(Valid), detector_block_v240/2(Valid), detector_block_v239/2(Valid), detector_block_v238/2(Valid), detector_block_v237/2(Valid), detector_block_v236/2(Valid), detector_block_v235/2(Valid), detector_block_v234/2(Valid), detector_block_v233/2(Valid), detector_block_v232/2(Valid), detector_block_v231/2(Valid), detector_block_v230/2(Valid), detector_block_v229/2(Valid), detector_block_v228/2(Valid), detector_block_v227/2(Valid), detector_block_v226/2(Valid), detector_block_v225/2(Valid), detector_block_v224/2(Valid), detector_block_v223/2(Valid), detector_block_v222/2(Valid), detector_block_v221/2(Valid), detector_block_v220/2(Valid), detector_block_v219/2(Valid), detector_block_v218/2(Valid), detector_block_v217/2(Valid), detector_block_v216/2(Valid), detector_block_v215/2(Valid), detector_block_v214/2(Valid), detector_block_v213/2(Valid), detector_block_v212/2(Valid), detector_block_v211/2(Valid), detector_block_v210/2(Valid), detector_block_v29/2(Valid), detector_block_v28/2(Valid), detector_block_v27/2(Valid), detector_block_v26/2(Valid), detector_block_v25/2(Valid), detector_block_v24/2(Valid), detector_block_v23/2(Valid), detector_block_v22/2(Valid), detector_block_v21/2(Valid), detector_block_v2/2(Valid)
  Counter/1 -> Slice1/1, Slice/1
  Slice/1 -> Mux1/1, Mux/1
  Mux2/1 -> Output/1
  Mux1/1 -> Mux2/3
  Mux/1 -> Mux2/2
  Slice1/1 -> Mux2/1
  detector_block_v263/1(Out1) -> Mux1/33
  detector_block_v262/1(Out1) -> Mux1/32
  detector_block_v261/1(Out1) -> Mux1/31
  detector_block_v260/1(Out1) -> Mux1/30
  detector_block_v259/1(Out1) -> Mux1/29
  detector_block_v258/1(Out1) -> Mux1/28
  detector_block_v257/1(Out1) -> Mux1/27
  detector_block_v256/1(Out1) -> Mux1/26
  detector_block_v255/1(Out1) -> Mux1/25
  detector_block_v254/1(Out1) -> Mux1/24
  detector_block_v253/1(Out1) -> Mux1/23
  detector_block_v252/1(Out1) -> Mux1/22
  detector_block_v251/1(Out1) -> Mux1/21
  detector_block_v250/1(Out1) -> Mux1/20
  detector_block_v249/1(Out1) -> Mux1/19
  detector_block_v248/1(Out1) -> Mux1/18
  detector_block_v247/1(Out1) -> Mux1/17
  detector_block_v246/1(Out1) -> Mux1/16
  detector_block_v245/1(Out1) -> Mux1/15
  detector_block_v244/1(Out1) -> Mux1/14
  detector_block_v243/1(Out1) -> Mux1/13
  detector_block_v242/1(Out1) -> Mux1/12
  detector_block_v241/1(Out1) -> Mux1/11
  detector_block_v240/1(Out1) -> Mux1/10
  detector_block_v239/1(Out1) -> Mux1/9
  detector_block_v238/1(Out1) -> Mux1/8
  detector_block_v237/1(Out1) -> Mux1/7
  detector_block_v236/1(Out1) -> Mux1/6
  detector_block_v235/1(Out1) -> Mux1/5
  detector_block_v234/1(Out1) -> Mux1/4
  detector_block_v233/1(Out1) -> Mux1/3
  detector_block_v232/1(Out1) -> Mux1/2
  detector_block_v231/1(Out1) -> Mux/33
  detector_block_v230/1(Out1) -> Mux/32
  detector_block_v229/1(Out1) -> Mux/31
  detector_block_v228/1(Out1) -> Mux/30
  detector_block_v227/1(Out1) -> Mux/29
  detector_block_v226/1(Out1) -> Mux/28
  detector_block_v225/1(Out1) -> Mux/27
  detector_block_v224/1(Out1) -> Mux/26
  detector_block_v223/1(Out1) -> Mux/25
  detector_block_v222/1(Out1) -> Mux/24
  detector_block_v221/1(Out1) -> Mux/23
  detector_block_v220/1(Out1) -> Mux/22
  detector_block_v219/1(Out1) -> Mux/21
  detector_block_v218/1(Out1) -> Mux/20
  detector_block_v217/1(Out1) -> Mux/19
  detector_block_v216/1(Out1) -> Mux/18
  detector_block_v215/1(Out1) -> Mux/17
  detector_block_v214/1(Out1) -> Mux/16
  detector_block_v213/1(Out1) -> Mux/15
  detector_block_v212/1(Out1) -> Mux/14
  detector_block_v211/1(Out1) -> Mux/13
  detector_block_v210/1(Out1) -> Mux/12
  detector_block_v29/1(Out1) -> Mux/11
  detector_block_v28/1(Out1) -> Mux/10
  detector_block_v27/1(Out1) -> Mux/9
  detector_block_v26/1(Out1) -> Mux/8
  detector_block_v25/1(Out1) -> Mux/7
  detector_block_v24/1(Out1) -> Mux/6
  detector_block_v23/1(Out1) -> Mux/5
  detector_block_v22/1(Out1) -> Mux/4
  detector_block_v21/1(Out1) -> Mux/3
  detector_block_v2/1(Out1) -> Mux/2
